simulink model "ebbers_moll_1"  (Simulink 7.4)
settings: Solver=ode23t  StartTime=0.0  StopTime=100e-6  MaxStep=1e-6  RelTol=1e-5
libraries: powerlib x18, simulink x2
settings Model: Creator=Dick Benson  LastModifiedBy=Dick
settings SolverCC: ZeroCrossControl=EnableAll
settings OptimizationCC: InlineInvariantSignals=on  InitFltsAndDblsToZero=on
settings DebuggingCC: SaveWithParameterizedLinksMsg=none  SignalResolutionControl=TryResolveAllWithWarning  MultiTaskDSMMsg=warning  MultiTaskCondExecSysMsg=none  StrictBusMsg=None
settings RTWCC: IncludeERTFirstTime=on
settings GRTTargetCC: TargetFcnLib=ansi_tfl_tmw.mat

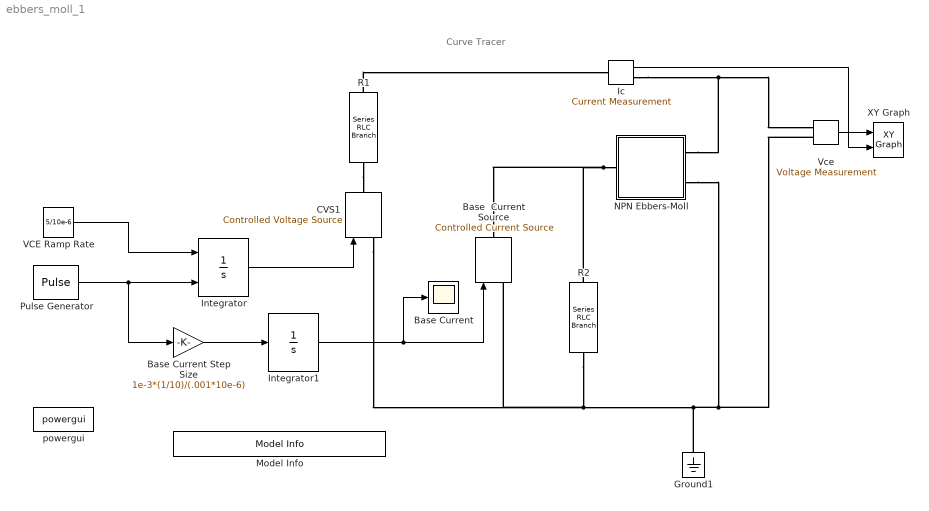
== system ebbers_moll_1 ==
  note: Curve Tracer
  Base  Current Source : powerlib/Electrical Sources/Controlled Current Source  DialogController=POWERSYS.PowerSysDialog  SystemSampleTime=-1  Initialize=on  Source_Type=AC  Amplitude=0  Phase=0  Frequency=0  Measurements=None
  Base Current : Scope
      settings: TimeRange=0.00012  YMin=0  YMax=0.0012  MaxDataPoints=50000
  Base Current Step Size : Gain  Gain=1e-3*(1/10)/(.001*10e-6)  ParameterDataType=sfix(16)  ParameterScaling=2^0  OutDataType=sfix(16)  OutScaling=2^0
  CVS1 : powerlib/Electrical Sources/Controlled Voltage Source  DialogController=POWERSYS.PowerSysDialog  SystemSampleTime=-1  Initialize=on  Source_Type=AC  Amplitude=0  Phase=0  Frequency=0  Measurements=None
  Ground1 : powerlib/Elements/Ground  DialogController=POWERSYS.PowerSysDialog  PhysicalDomain=powersysdomain  SubClassName=unknown  LeftPortType=p1  RightPortType=p1  LConnTagsString=a
  "Ic " : powerlib/Measurements/Current Measurement  DialogController=POWERSYS.PowerSysDialog  SystemSampleTime=-1  PhasorSimulation=off  OutputType=Complex  PSBequivalent=0
  Integrator : Integrator  ExternalReset=falling
  Integrator1 : Integrator
  Model Info : simulink/Model-Wide Utilities/Model Info  SystemSampleTime=-1  InitialBlockCM=None  BlockCM=None  Frame=on  DisplayStringWithTags=Copywrite 2005-2010 The MathWorks, Inc.  HorizontalTextAlignment=Center  LeftAlignmentValue=0.5  SourceBlockDiagram=ebbers_moll_1  TagMaxNumber=20
  "NPN Ebbers-Moll " : Subsystem  mask{Beta=100, IEs=1e-8;, ICs=1e-8;, Ro=1e3, Cbc=5e-12, Cbe=50e-12, Rbb=100}
      mask init:
      | k = 1.38e-23;
      | q = 1.6e-19;
      | T = 290;
      | Vt = k*T/q;
  Pulse Generator : DiscretePulseGenerator  PulseType=Time based  Amplitude=1  Period=10e-6  PulseWidth=0.1  PhaseDelay=0  SampleTime=1
  R1 : powerlib/Elements/Series RLC Branch  DialogController=POWERSYS.PowerSysDialog  PhysicalDomain=powersysdomain  SubClassName=unknown  LeftPortType=p1  RightPortType=p1  LConnTagsString=__new0  RConnTagsString=__new0  BranchType=R  Resistance=1  Inductance=1.0  SetiL0=off  InitialCurrent=0  Capacitance=1.0  Setx0=off  InitialVoltage=0  Measurements=None
  R2 : powerlib/Elements/Series RLC Branch  DialogController=POWERSYS.PowerSysDialog  PhysicalDomain=powersysdomain  SubClassName=unknown  LeftPortType=p1  RightPortType=p1  LConnTagsString=__new0  RConnTagsString=__new0  BranchType=R  Resistance=100000  Inductance=1.0  SetiL0=off  InitialCurrent=0  Capacitance=1.0  Setx0=off  InitialVoltage=0  Measurements=None
  VCE Ramp Rate : Constant  Value=5/10e-6  OutDataType=sfix(16)  OutScaling=2^0
  "Vce " : powerlib/Measurements/Voltage Measurement  DialogController=POWERSYS.PowerSysDialog  SystemSampleTime=-1  PhasorSimulation=off  OutputType=Complex  PSBequivalent=0
  XY Graph : simulink/Sinks/XY Graph  SystemSampleTime=-1  xmin=0  xmax=4  ymin=0  ymax=.1  st=-1
  powergui : powerlib/powergui  SystemSampleTime=-1  SimulationMode=Continuous  SampleTime=0  frequency=60  SPID=off  DisableSnubberDevices=off  DisableRonSwitches=off  DisableVfSwitches=off  SwTol=0  Interpol=off  frequencyindice=0  echomessages=off  HookPort=off  DisplayEquations=off  FunctionMessages=off  EnableUseOfTLC=off  x0status=blocks  RestoreLinks=warning  Frange=[0:2:500]  Ylog=off  Xlog=on  ShowGrid=off  save=off  variable=ZData  ZoomFFT=on  StartTime=0.0  cycles=1  DisplayStyle=1  fundamental=60  FreqAxis=off  MaxFrequency=1000  frequencyindicesteady=1  RmsSteady=1  display=off  Ts=0  methode=off
  wires:
  "Vce "/1 -> XY Graph/1
  Integrator1/1 -> Base  Current Source/1, Base Current/1
  "Ic "/1 -> XY Graph/2
  VCE Ramp Rate/1 -> Integrator/1
  Pulse Generator/1 -> Integrator/2, Base Current Step Size/1
  Integrator/1 -> CVS1/1
  Base Current Step Size/1 -> Integrator1/1
  connections:
  "NPN Ebbers-Moll "/RConn2 -- "Vce "/LConn2 -- Ground1/LConn1 -- CVS1/LConn1 -- Base  Current Source/LConn1 -- R2/RConn1
  "NPN Ebbers-Moll "/LConn1 -- R2/LConn1 -- Base  Current Source/RConn1
  "NPN Ebbers-Moll "/RConn1 -- "Vce "/LConn1 -- "Ic "/RConn1
  R1/RConn1 -- CVS1/RConn1
  R1/LConn1 -- "Ic "/LConn1

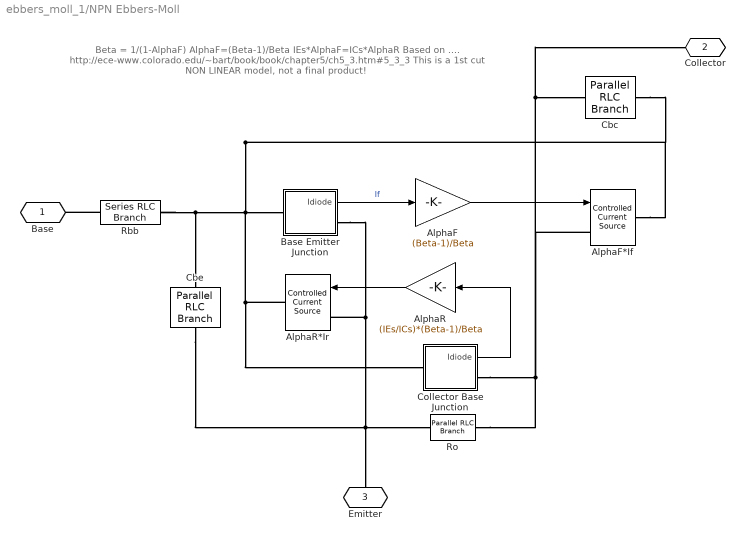
== system ebbers_moll_1/NPN Ebbers-Moll  ==
  note: Beta = 1/(1-AlphaF)
      | AlphaF=(Beta-1)/Beta
      | IEs*AlphaF=ICs*AlphaR
      |
      | Based on ....
      | http://ece-www.colorado.edu/~bart/book/book/chapter5/ch5_3.htm#5_3_3
      |
      | This is a 1st cut NON LINEAR model, not a final product!
  AlphaF : Gain  Gain=(Beta-1)/Beta  ParameterDataType=sfix(16)  ParameterScaling=2^0  OutDataType=sfix(16)  OutScaling=2^0
  AlphaF*If : powerlib/Electrical Sources/Controlled Current Source  Description=source block  DialogController=POWERSYS.PowerSysDialog  SystemSampleTime=-1  Initialize=off  Source_Type=AC  Amplitude=-0.025  Phase=0  Frequency=0  Measurements=None
      settings: AttributesFormatString=\n
  AlphaR : Gain  Gain=(IEs/ICs)*(Beta-1)/Beta  ParameterDataType=sfix(16)  ParameterScaling=2^0  OutDataType=sfix(16)  OutScaling=2^0
  AlphaR*Ir : powerlib/Electrical Sources/Controlled Current Source  Description=source block  DialogController=POWERSYS.PowerSysDialog  SystemSampleTime=-1  Initialize=off  Source_Type=AC  Amplitude=-0.025  Phase=0  Frequency=0  Measurements=None
      settings: AttributesFormatString=\n
  Base Emitter Junction : Subsystem  AncestorBlock=simcircuits_library_1/diode  mask{Is=IEs}
      mask prompts: Is "Saturation Current"
      mask Display: plot(-140,-140,150,140,2*[30,30,59,30,30,0]-75,(2*[71,50,72,92,71,71]-92),2*[59,59]-75,(2*[50,93]-92),[116,59]-16,(2*[71,71]-90));
  Cbc : powerlib/Elements/Parallel RLC Branch  DialogController=POWERSYS.PowerSysDialog  PhysicalDomain=powersysdomain  SubClassName=unknown  LeftPortType=p1  RightPortType=p1  LConnTagsString=a  RConnTagsString=__new0  BranchType=C  Resistance=1.0  Inductance=1.0  SetiL0=off  InitialCurrent=0  Capacitance=Cbc  Setx0=off  InitialVoltage=0  Measurements=None
  Cbe : powerlib/Elements/Parallel RLC Branch  DialogController=POWERSYS.PowerSysDialog  PhysicalDomain=powersysdomain  SubClassName=unknown  LeftPortType=p1  RightPortType=p1  LConnTagsString=a  RConnTagsString=__new0  BranchType=C  Resistance=1.0  Inductance=1.0  SetiL0=off  InitialCurrent=0  Capacitance=Cbe  Setx0=off  InitialVoltage=0  Measurements=None
  Collector Base Junction : Subsystem  AncestorBlock=simcircuits_library_1/diode  mask{Is=ICs}
      mask prompts: Is "Saturation Current"
      mask Display: plot(-140,-140,150,140,2*[30,30,59,30,30,0]-75,(2*[71,50,72,92,71,71]-92),2*[59,59]-75,(2*[50,93]-92),[116,59]-16,(2*[71,71]-90));
  Rbb : powerlib/Elements/Series RLC Branch  DialogController=POWERSYS.PowerSysDialog  PhysicalDomain=powersysdomain  SubClassName=unknown  LeftPortType=p1  RightPortType=p1  LConnTagsString=__new0  RConnTagsString=__new0  BranchType=R  Resistance=Rbb  Inductance=1.0  SetiL0=off  InitialCurrent=0  Capacitance=1.0  Setx0=off  InitialVoltage=0  Measurements=None
  Ro : powerlib/Elements/Parallel RLC Branch  DialogController=POWERSYS.PowerSysDialog  PhysicalDomain=powersysdomain  SubClassName=unknown  LeftPortType=p1  RightPortType=p1  LConnTagsString=a  RConnTagsString=__new0  BranchType=R  Resistance=Ro  Inductance=1.0  SetiL0=off  InitialCurrent=0  Capacitance=1.0  Setx0=off  InitialVoltage=0  Measurements=None
  Base : PMIOPort  Port=1  Side=Left
  Collector : PMIOPort  Port=2  Side=Right
  Emitter : PMIOPort  Port=3  Side=Right
  wires:
  Base Emitter Junction/1(Idiode) -> AlphaF/1  "If"
  AlphaF/1 -> AlphaF*If/1
  Collector Base Junction/1(Idiode) -> AlphaR/1
  AlphaR/1 -> AlphaR*Ir/1
  connections:
  Rbb/RConn1 -- Cbe/LConn1 -- Base Emitter Junction/LConn1 -- AlphaF*If/RConn1 -- Cbc/RConn1 -- AlphaR*Ir/RConn1 -- Collector Base Junction/LConn1
  AlphaR*Ir/LConn1 -- Emitter/RConn1 -- Cbe/RConn1 -- Ro/LConn1 -- Base Emitter Junction/RConn1
  AlphaF*If/LConn1 -- Collector/RConn1 -- Cbc/LConn1 -- Collector Base Junction/RConn1 -- Ro/RConn1
  Rbb/LConn1 -- Base/RConn1

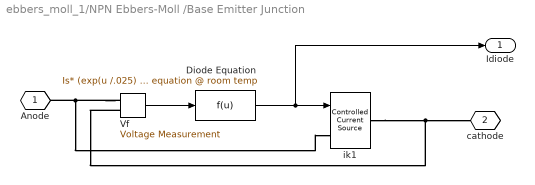
== system ebbers_moll_1/NPN Ebbers-Moll /Base Emitter Junction ==
  Diode Equation : Fcn  Expr="Is* (exp(u /.025)  -1  );  % ideal diode equation @ room temp"
  "Vf " : powerlib/Measurements/Voltage Measurement  Tag=PoWeRsYsTeMmEaSuReMeNt  DialogController=POWERSYS.PowerSysDialog  SystemSampleTime=-1  PhasorSimulation=off  OutputType=Magnitude  PSBequivalent=0
  ik1 : powerlib/Electrical Sources/Controlled Current Source  Description=source block  DialogController=POWERSYS.PowerSysDialog  SystemSampleTime=-1  Initialize=on  Source_Type=AC  Amplitude=0  Phase=0  Frequency=0  Measurements=None
      settings: AttributesFormatString=\n
  Anode : PMIOPort  Tag=PMCPort  Port=1  Side=Left
  "cathode " : PMIOPort  Tag=PMCPort  Port=2  Side=Right
  Idiode : Outport  OutDataType=sfix(16)  OutScaling=2^0
  wires:
  "Vf "/1 -> Diode Equation/1
  Diode Equation/1 -> ik1/1, Idiode/1
  connections:
  "Vf "/LConn1 -- Anode/RConn1 -- ik1/LConn1
  "Vf "/LConn2 -- "cathode "/RConn1 -- ik1/RConn1

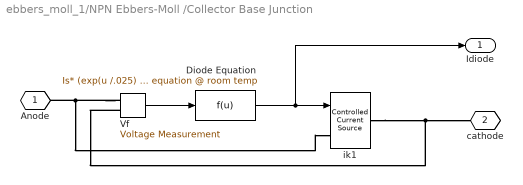
== system ebbers_moll_1/NPN Ebbers-Moll /Collector Base Junction ==
  Diode Equation : Fcn  Expr="Is* (exp(u /.025)  -1  );  % ideal diode equation @ room temp"
  "Vf " : powerlib/Measurements/Voltage Measurement  Tag=PoWeRsYsTeMmEaSuReMeNt  DialogController=POWERSYS.PowerSysDialog  SystemSampleTime=-1  PhasorSimulation=off  OutputType=Magnitude  PSBequivalent=0
  ik1 : powerlib/Electrical Sources/Controlled Current Source  Description=source block  DialogController=POWERSYS.PowerSysDialog  SystemSampleTime=-1  Initialize=on  Source_Type=AC  Amplitude=0  Phase=0  Frequency=0  Measurements=None
      settings: AttributesFormatString=\n
  Anode : PMIOPort  Tag=PMCPort  Port=1  Side=Left
  "cathode " : PMIOPort  Tag=PMCPort  Port=2  Side=Right
  Idiode : Outport  OutDataType=sfix(16)  OutScaling=2^0
  wires:
  Diode Equation/1 -> Idiode/1, ik1/1
  "Vf "/1 -> Diode Equation/1
  connections:
  ik1/RConn1 -- "cathode "/RConn1 -- "Vf "/LConn2
  ik1/LConn1 -- Anode/RConn1 -- "Vf "/LConn1
